simulink model "quad_linear_model"  (R2024b)
settings: Solver=FixedStepDiscrete  StartTime=0.0  StopTime=10.0  FixedStep=0.010000  RelTol=1e-3
model workspace (MAT data in the model file):
  already_pp = 1
values from neighbouring files (symbols this model uses):
  Ts = 0.01    [quadcopterParameters.m]
undefined symbols (not defined in the file or in its folder): s_alt, s_att_x
settings Model: Creator=elia  LastModifiedBy=elia
settings DebuggingCC: AlgebraicLoopMsg=error  ArtificialAlgebraicLoopMsg=error  SaveWithDisabledLinksMsg=none  SingleTaskRateTransMsg=error

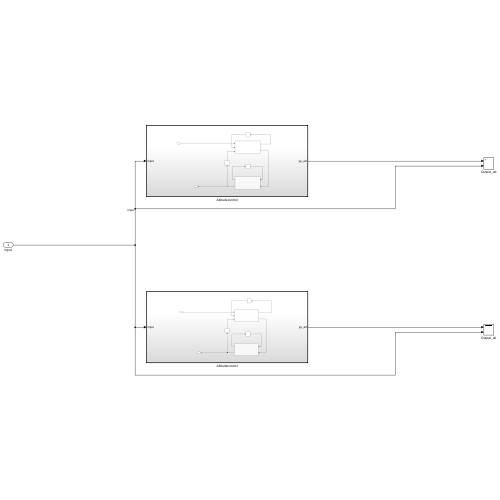
[thumbnail: Simulink's stored preview of the top-level diagram]
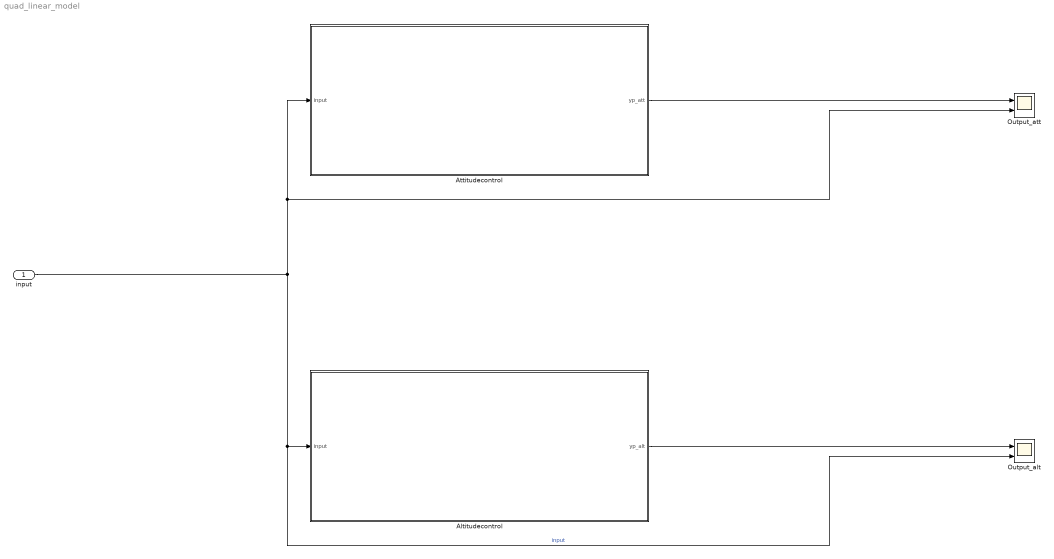
== system quad_linear_model ==
  input : Inport
  Altitudecontrol : Subsystem  TreatAsAtomicUnit=on
  Attitudecontrol : Subsystem  TreatAsAtomicUnit=on
  Output_alt : Scope  NumInputPorts=2
  Output_att : Scope  NumInputPorts=2
  wires:
  Attitudecontrol/1(yp_att) -> Output_att/1
  Altitudecontrol/1(yp_alt) -> Output_alt/1
  input/1 -> Altitudecontrol/1(input), Output_alt/2, Attitudecontrol/1(input), Output_att/2  "input"

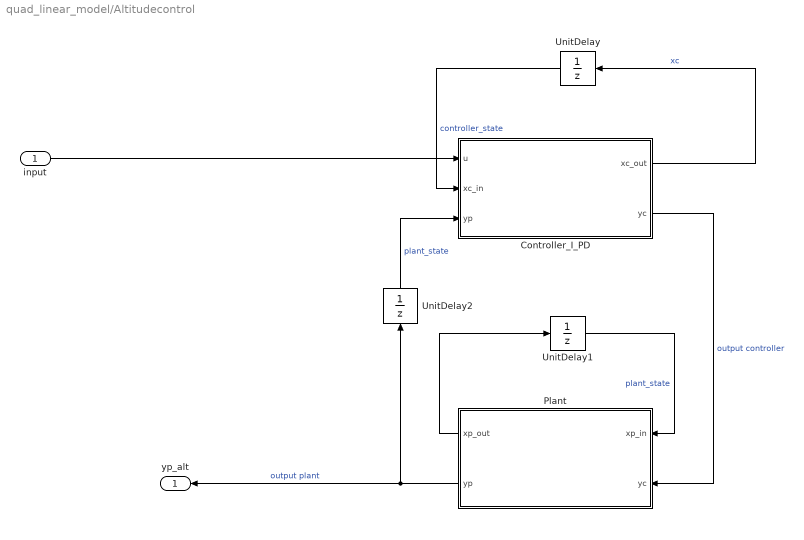
== system quad_linear_model/Altitudecontrol ==
  input : Inport
  Controller_I_PD : Subsystem  TreatAsAtomicUnit=on
  Plant : Subsystem  TreatAsAtomicUnit=on
  UnitDelay : UnitDelay  SampleTime=Ts  HasFrameUpgradeWarning=on
  UnitDelay1 : UnitDelay  SampleTime=Ts  HasFrameUpgradeWarning=on
  UnitDelay2 : UnitDelay  SampleTime=Ts  HasFrameUpgradeWarning=on
  yp_alt : Outport
  wires:
  Plant/2(yp) -> yp_alt/1, UnitDelay2/1  "output plant"
  Plant/1(xp_out) -> UnitDelay1/1
  UnitDelay1/1 -> Plant/1(xp_in)  "plant_state"
  UnitDelay/1 -> Controller_I_PD/2(xc_in)  "controller_state"
  Controller_I_PD/2(yc) -> Plant/2(yc)  "output controller"
  Controller_I_PD/1(xc_out) -> UnitDelay/1  "xc"
  input/1 -> Controller_I_PD/1(u)
  UnitDelay2/1 -> Controller_I_PD/3(yp)  "plant_state"

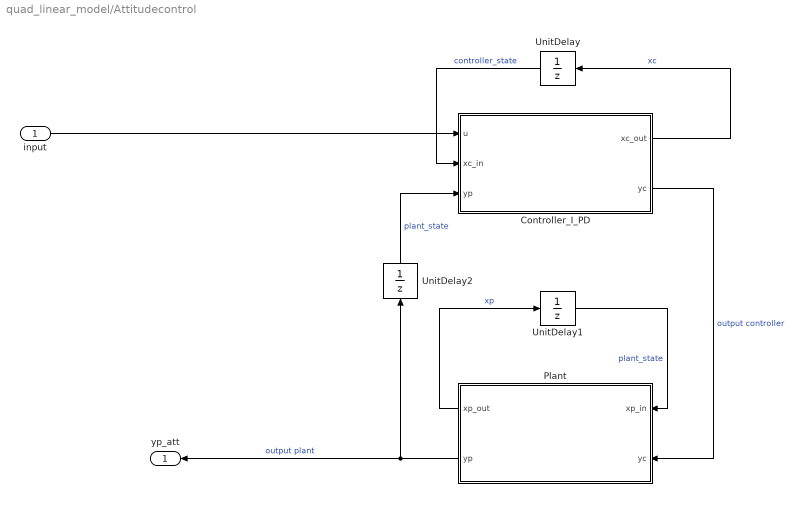
== system quad_linear_model/Attitudecontrol ==
  input : Inport
  Controller_I_PD : Subsystem  TreatAsAtomicUnit=on
  Plant : Subsystem  TreatAsAtomicUnit=on
  UnitDelay : UnitDelay  SampleTime=Ts  HasFrameUpgradeWarning=on
  UnitDelay1 : UnitDelay  SampleTime=Ts  HasFrameUpgradeWarning=on
  UnitDelay2 : UnitDelay  SampleTime=Ts  HasFrameUpgradeWarning=on
  yp_att : Outport
  wires:
  Plant/2(yp) -> UnitDelay2/1, yp_att/1  "output plant"
  Plant/1(xp_out) -> UnitDelay1/1  "xp"
  UnitDelay1/1 -> Plant/1(xp_in)  "plant_state"
  UnitDelay/1 -> Controller_I_PD/2(xc_in)  "controller_state"
  Controller_I_PD/2(yc) -> Plant/2(yc)  "output controller"
  Controller_I_PD/1(xc_out) -> UnitDelay/1  "xc"
  input/1 -> Controller_I_PD/1(u)
  UnitDelay2/1 -> Controller_I_PD/3(yp)  "plant_state"

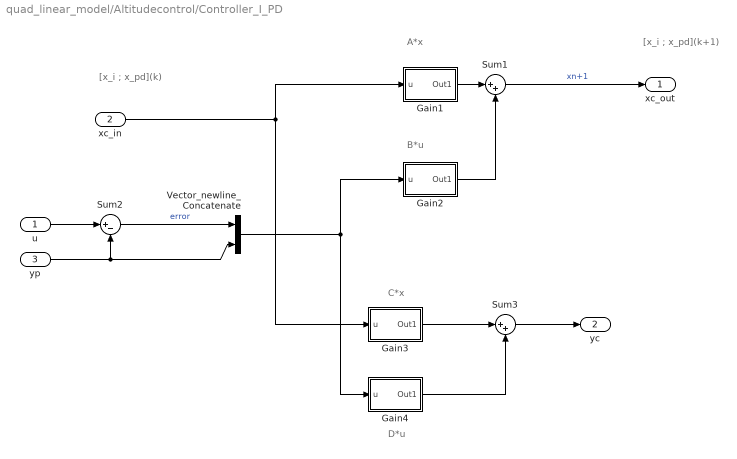
== system quad_linear_model/Altitudecontrol/Controller_I_PD ==
  note: C*x
  note: B*u
  note: A*x
  note: [x_i ;
      | x_pd](k+1)
  note: [x_i ;
      | x_pd](k)
  note: D*u
  u : Inport
  xc_in : Inport  Port=2
  yp : Inport  Port=3
  Gain1 : Subsystem  TreatAsAtomicUnit=on
  Gain2 : Subsystem  TreatAsAtomicUnit=on
  Gain3 : Subsystem  TreatAsAtomicUnit=on
  Gain4 : Subsystem  TreatAsAtomicUnit=on
  Sum1 : Sum  Inputs=|++
  Sum2 : Sum  Inputs=|+-
  Sum3 : Sum  Inputs=|++
  Vector_newline_Concatenate : Concatenate
  xc_out : Outport
  yc : Outport  Port=2
  wires:
  Gain2/1(Out1) -> Sum1/2
  Sum1/1 -> xc_out/1  "xn+1"
  yp/1 -> Vector_newline_Concatenate/2, Sum2/2
  Sum3/1 -> yc/1
  u/1 -> Sum2/1
  Gain1/1(Out1) -> Sum1/1
  xc_in/1 -> Gain3/1(u), Gain1/1(u)
  Vector_newline_Concatenate/1 -> Gain4/1(u), Gain2/1(u)
  Sum2/1 -> Vector_newline_Concatenate/1  "error"
  Gain4/1(Out1) -> Sum3/2
  Gain3/1(Out1) -> Sum3/1

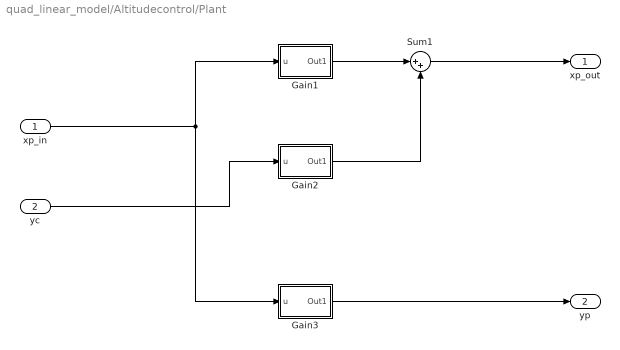
== system quad_linear_model/Altitudecontrol/Plant ==
  xp_in : Inport
  yc : Inport  Port=2
  Gain1 : Subsystem  TreatAsAtomicUnit=on
  Gain2 : Subsystem  TreatAsAtomicUnit=on
  Gain3 : Subsystem  TreatAsAtomicUnit=on
  Sum1 : Sum  Inputs=|++
  xp_out : Outport
  yp : Outport  Port=2
  wires:
  xp_in/1 -> Gain1/1(u), Gain3/1(u)
  Gain1/1(Out1) -> Sum1/1
  Gain2/1(Out1) -> Sum1/2
  yc/1 -> Gain2/1(u)
  Sum1/1 -> xp_out/1
  Gain3/1(Out1) -> yp/1

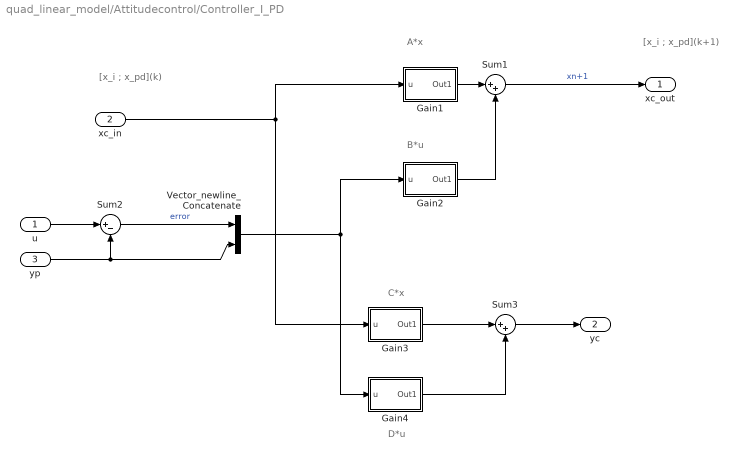
== system quad_linear_model/Attitudecontrol/Controller_I_PD ==
  note: C*x
  note: B*u
  note: A*x
  note: [x_i ;
      | x_pd](k+1)
  note: [x_i ;
      | x_pd](k)
  note: D*u
  u : Inport
  xc_in : Inport  Port=2
  yp : Inport  Port=3
  Gain1 : Subsystem  TreatAsAtomicUnit=on
  Gain2 : Subsystem  TreatAsAtomicUnit=on
  Gain3 : Subsystem  TreatAsAtomicUnit=on
  Gain4 : Subsystem  TreatAsAtomicUnit=on
  Sum1 : Sum  Inputs=|++
  Sum2 : Sum  Inputs=|+-
  Sum3 : Sum  Inputs=|++
  Vector_newline_Concatenate : Concatenate
  xc_out : Outport
  yc : Outport  Port=2
  wires:
  Gain2/1(Out1) -> Sum1/2
  Sum1/1 -> xc_out/1  "xn+1"
  yp/1 -> Vector_newline_Concatenate/2, Sum2/2
  Sum3/1 -> yc/1
  u/1 -> Sum2/1
  Gain1/1(Out1) -> Sum1/1
  xc_in/1 -> Gain3/1(u), Gain1/1(u)
  Vector_newline_Concatenate/1 -> Gain4/1(u), Gain2/1(u)
  Sum2/1 -> Vector_newline_Concatenate/1  "error"
  Gain4/1(Out1) -> Sum3/2
  Gain3/1(Out1) -> Sum3/1

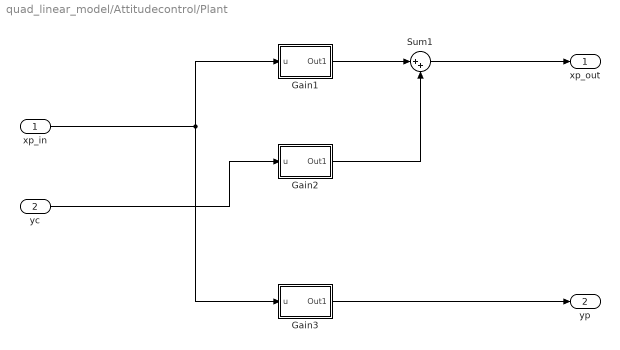
== system quad_linear_model/Attitudecontrol/Plant ==
  xp_in : Inport
  yc : Inport  Port=2
  Gain1 : Subsystem  TreatAsAtomicUnit=on
  Gain2 : Subsystem  TreatAsAtomicUnit=on
  Gain3 : Subsystem  TreatAsAtomicUnit=on
  Sum1 : Sum  Inputs=|++
  xp_out : Outport
  yp : Outport  Port=2
  wires:
  xp_in/1 -> Gain1/1(u), Gain3/1(u)
  Gain1/1(Out1) -> Sum1/1
  Gain2/1(Out1) -> Sum1/2
  yc/1 -> Gain2/1(u)
  Sum1/1 -> xp_out/1
  Gain3/1(Out1) -> yp/1

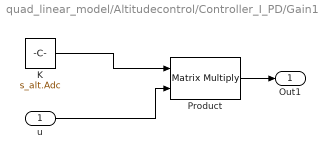
== system quad_linear_model/Altitudecontrol/Controller_I_PD/Gain1 ==
  u : Inport  OutDataTypeStr=double
  K : Constant  Value=s_alt.Adc  VectorParams1D=off
  Product : Product  Multiplication=Matrix(*)
  Out1 : Outport  VectorParamsAs1DForOutWhenUnconnected=off
  wires:
  Product/1 -> Out1/1
  K/1 -> Product/1
  u/1 -> Product/2

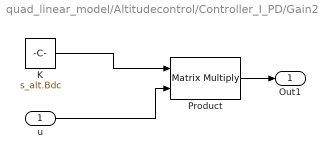
== system quad_linear_model/Altitudecontrol/Controller_I_PD/Gain2 ==
  u : Inport  OutDataTypeStr=double
  K : Constant  Value=s_alt.Bdc  VectorParams1D=off
  Product : Product  Multiplication=Matrix(*)
  Out1 : Outport  VectorParamsAs1DForOutWhenUnconnected=off
  wires:
  Product/1 -> Out1/1
  K/1 -> Product/1
  u/1 -> Product/2

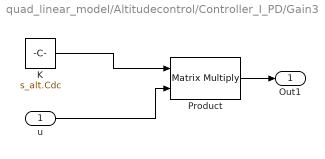
== system quad_linear_model/Altitudecontrol/Controller_I_PD/Gain3 ==
  u : Inport  OutDataTypeStr=double
  K : Constant  Value=s_alt.Cdc  VectorParams1D=off
  Product : Product  Multiplication=Matrix(*)
  Out1 : Outport  VectorParamsAs1DForOutWhenUnconnected=off
  wires:
  Product/1 -> Out1/1
  K/1 -> Product/1
  u/1 -> Product/2

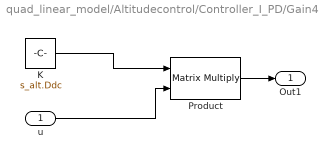
== system quad_linear_model/Altitudecontrol/Controller_I_PD/Gain4 ==
  u : Inport  OutDataTypeStr=double
  K : Constant  Value=s_alt.Ddc  VectorParams1D=off
  Product : Product  Multiplication=Matrix(*)
  Out1 : Outport  VectorParamsAs1DForOutWhenUnconnected=off
  wires:
  Product/1 -> Out1/1
  K/1 -> Product/1
  u/1 -> Product/2

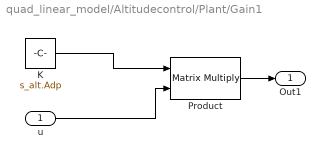
== system quad_linear_model/Altitudecontrol/Plant/Gain1 ==
  u : Inport  OutDataTypeStr=double
  K : Constant  Value=s_alt.Adp  VectorParams1D=off
  Product : Product  Multiplication=Matrix(*)
  Out1 : Outport  VectorParamsAs1DForOutWhenUnconnected=off
  wires:
  Product/1 -> Out1/1
  K/1 -> Product/1
  u/1 -> Product/2

== system quad_linear_model/Altitudecontrol/Plant/Gain2 ==
  u : Inport  OutDataTypeStr=double
  K : Constant  Value=s_alt.Bdp  VectorParams1D=off
  Product : Product  Multiplication=Matrix(*)
  Out1 : Outport  VectorParamsAs1DForOutWhenUnconnected=off
  wires:
  Product/1 -> Out1/1
  K/1 -> Product/1
  u/1 -> Product/2

== system quad_linear_model/Altitudecontrol/Plant/Gain3 ==
  u : Inport  OutDataTypeStr=double
  K : Constant  Value=s_alt.Cdp  VectorParams1D=off
  Product : Product  Multiplication=Matrix(*)
  Out1 : Outport  VectorParamsAs1DForOutWhenUnconnected=off
  wires:
  Product/1 -> Out1/1
  K/1 -> Product/1
  u/1 -> Product/2

== system quad_linear_model/Attitudecontrol/Controller_I_PD/Gain1 ==
  u : Inport  OutDataTypeStr=double
  K : Constant  Value=s_att_x.Adc  VectorParams1D=off
  Product : Product  Multiplication=Matrix(*)
  Out1 : Outport  VectorParamsAs1DForOutWhenUnconnected=off
  wires:
  Product/1 -> Out1/1
  K/1 -> Product/1
  u/1 -> Product/2

== system quad_linear_model/Attitudecontrol/Controller_I_PD/Gain2 ==
  u : Inport  OutDataTypeStr=double
  K : Constant  Value=s_att_x.Bdc  VectorParams1D=off
  Product : Product  Multiplication=Matrix(*)
  Out1 : Outport  VectorParamsAs1DForOutWhenUnconnected=off
  wires:
  Product/1 -> Out1/1
  K/1 -> Product/1
  u/1 -> Product/2

== system quad_linear_model/Attitudecontrol/Controller_I_PD/Gain3 ==
  u : Inport  OutDataTypeStr=double
  K : Constant  Value=s_att_x.Cdc  VectorParams1D=off
  Product : Product  Multiplication=Matrix(*)
  Out1 : Outport  VectorParamsAs1DForOutWhenUnconnected=off
  wires:
  Product/1 -> Out1/1
  K/1 -> Product/1
  u/1 -> Product/2

== system quad_linear_model/Attitudecontrol/Controller_I_PD/Gain4 ==
  u : Inport  OutDataTypeStr=double
  K : Constant  Value=s_att_x.Ddc  VectorParams1D=off
  Product : Product  Multiplication=Matrix(*)
  Out1 : Outport  VectorParamsAs1DForOutWhenUnconnected=off
  wires:
  Product/1 -> Out1/1
  K/1 -> Product/1
  u/1 -> Product/2

== system quad_linear_model/Attitudecontrol/Plant/Gain1 ==
  u : Inport  OutDataTypeStr=double
  K : Constant  Value=s_att_x.Adp  VectorParams1D=off
  Product : Product  Multiplication=Matrix(*)
  Out1 : Outport  VectorParamsAs1DForOutWhenUnconnected=off
  wires:
  Product/1 -> Out1/1
  K/1 -> Product/1
  u/1 -> Product/2

== system quad_linear_model/Attitudecontrol/Plant/Gain2 ==
  u : Inport  OutDataTypeStr=double
  K : Constant  Value=s_att_x.Bdp  VectorParams1D=off
  Product : Product  Multiplication=Matrix(*)
  Out1 : Outport  VectorParamsAs1DForOutWhenUnconnected=off
  wires:
  Product/1 -> Out1/1
  K/1 -> Product/1
  u/1 -> Product/2

== system quad_linear_model/Attitudecontrol/Plant/Gain3 ==
  u : Inport  OutDataTypeStr=double
  K : Constant  Value=s_att_x.Cdp  VectorParams1D=off
  Product : Product  Multiplication=Matrix(*)
  Out1 : Outport  VectorParamsAs1DForOutWhenUnconnected=off
  wires:
  Product/1 -> Out1/1
  K/1 -> Product/1
  u/1 -> Product/2
